simulink model "RT_ueb7_a2"  (R2013a)
settings: Solver=ode45  StartTime=0.0  StopTime=10.0  RelTol=1e-3
values from neighbouring files (symbols this model uses):
  alpha = 2    [RT_wok_aufgabe.m]    (also in servo_2_proc.m = alpha_calc; servo_3_proc.m = alpha_calc)
  K = Kk(i)    [RT_wok_aufgabe.m]    (also in nyquist_stabil.m = 0.2; s_schrittantwort.m = 1; servo_4_proc.m = 1)
settings Model: Creator=mainster  LastModifiedBy=mainster
settings DebuggingCC: SolverPrmCheckMsg=none

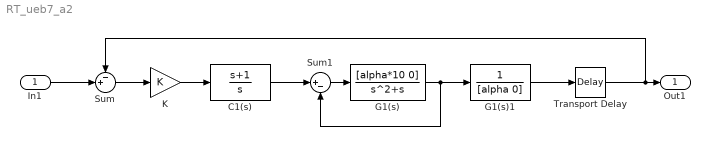
== system RT_ueb7_a2 ==
  In1 : Inport
  C1(s) : TransferFcn  Numerator=[1 1]  Denominator=[1 0]
  G1(s) : TransferFcn  Numerator=[alpha*10 0]  Denominator=[1 1 0]
  G1(s)1 : TransferFcn  Denominator=[alpha 0]
  K : Gain  Gain=K
  Sum : Sum  Inputs=-+|
  Sum1 : Sum  Inputs=|+-
  Transport Delay : TransportDelay
  Out1 : Outport
  wires:
  Sum/1 -> K/1
  K/1 -> C1(s)/1
  C1(s)/1 -> Sum1/1
  Sum1/1 -> G1(s)/1
  G1(s)/1 -> Sum1/2, G1(s)1/1
  In1/1 -> Sum/2
  G1(s)1/1 -> Transport Delay/1
  Transport Delay/1 -> Sum/1, Out1/1
